simulink model "quadrotor_3dof_fas1"  (R2024a)
settings: Solver=VariableStepAuto  StartTime=0.0  StopTime=20  FixedStep=0.0025  RelTol=1e-3
settings Model: SimulationMode=accelerator  Creator=Dell  LastModifiedBy=44915
settings RTWCC: GPUComputeCapability=3.5

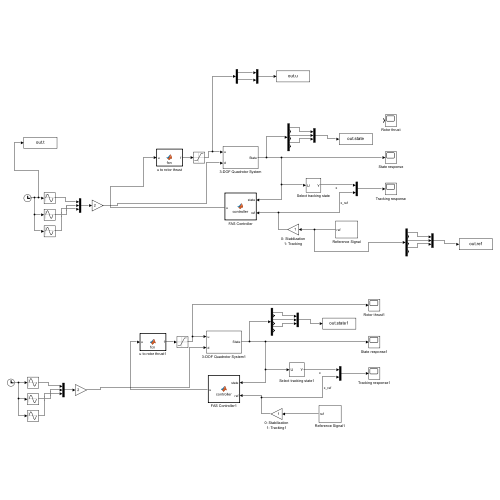
[thumbnail: Simulink's stored preview of the top-level diagram]
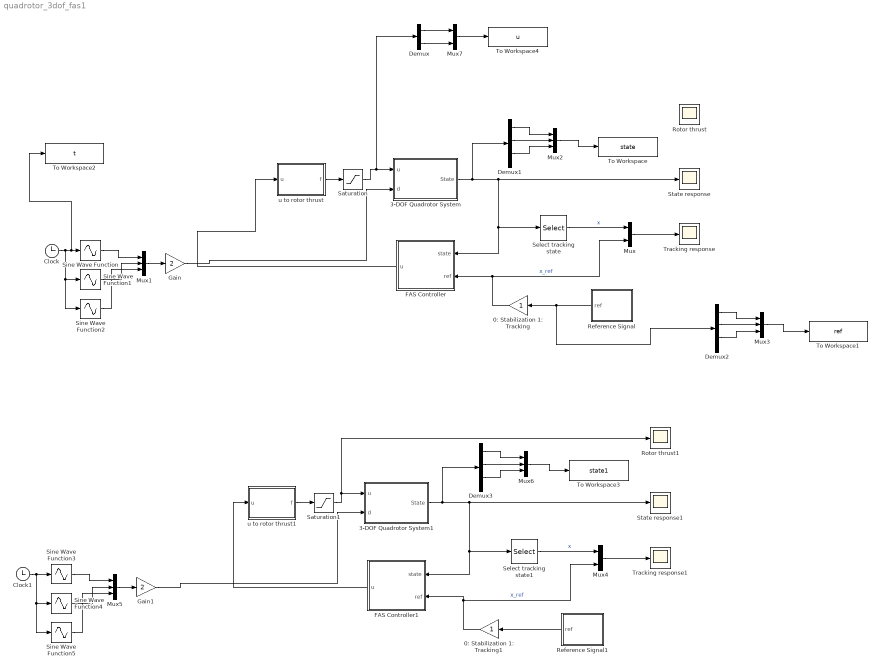
== system quadrotor_3dof_fas1 ==
  0: Stabilization 1: Tracking : Gain
  0: Stabilization 1: Tracking1 : Gain
  3-DOF Quadrotor System : Subsystem
  3-DOF Quadrotor System1 : Subsystem
  Clock : Clock
  Clock1 : Clock
  Demux : Demux  Outputs=2
  Demux1 : Demux  Outputs=6
  Demux2 : Demux  Outputs=6
  Demux3 : Demux  Outputs=6
  FAS Controller : MATLAB Function  TreatAsAtomicUnit=on
  FAS Controller1 : MATLAB Function  TreatAsAtomicUnit=on
  Gain : Gain  Gain=2
  Gain1 : Gain  Gain=2
  Mux : Mux  Inputs=2
  Mux{1..3,5..6} (5 alike) : Mux  Inputs=3
  Mux4 : Mux  Inputs=2
  Mux7 : Mux  Inputs=2
  Reference Signal : Subsystem
  Reference Signal1 : Subsystem
  Rotor thrust : Scope
  Rotor thrust1 : Scope
  Saturation : Saturate  UpperLimit=50  LowerLimit=-50
  Saturation1 : Saturate  UpperLimit=50  LowerLimit=-50
  Select tracking state : Selector  InputPortWidth=6  IndexOptions=Index vector (dialog)  Indices=[1]  OutputSizes=1
  Select tracking state1 : Selector  InputPortWidth=6  IndexOptions=Index vector (dialog)  Indices=[1]  OutputSizes=1
  Sine Wave Function{,1..5} (6 alike) : Sin  TimeSource=Use external signal  Amplitude=0.01  SampleTime=0
  State response : Scope
  State response1 : Scope
  To Workspace : ToWorkspace  VariableName=state  SampleTime=-1
  To Workspace1 : ToWorkspace  VariableName=ref  SampleTime=-1
  To Workspace2 : ToWorkspace  VariableName=t  SampleTime=-1
  To Workspace3 : ToWorkspace  VariableName=state1  SampleTime=-1
  To Workspace4 : ToWorkspace  VariableName=u  SampleTime=-1
  Tracking response : Scope
  Tracking response1 : Scope
  u to rotor thrust : MATLAB Function  TreatAsAtomicUnit=on
  u to rotor thrust1 : MATLAB Function  TreatAsAtomicUnit=on
  wires:
  3-DOF Quadrotor System/1(State) -> Demux1/1, State response/1, Select tracking state/1, FAS Controller/1(state)
  u to rotor thrust/1(f) -> Saturation/1
  Select tracking state/1 -> Mux/1  "x"
  Mux/1 -> Tracking response/1
  0: Stabilization 1: Tracking/1 -> Mux/2, FAS Controller/2(ref)  "x_ref"
  Reference Signal/1(ref) -> Demux2/1, 0: Stabilization 1: Tracking/1
  Saturation/1 -> Demux/1, 3-DOF Quadrotor System/1(u)
  Clock/1 -> Sine Wave Function2/1, Sine Wave Function1/1, To Workspace2/1, Sine Wave Function/1
  Sine Wave Function/1 -> Mux1/1
  Sine Wave Function1/1 -> Mux1/2
  Sine Wave Function2/1 -> Mux1/3
  Mux1/1 -> Gain/1
  Demux1/1 -> Mux2/1
  Demux1/3 -> Mux2/2
  Demux1/5 -> Mux2/3
  Mux2/1 -> To Workspace/1
  Demux2/3 -> Mux3/2
  Demux2/5 -> Mux3/3
  Demux2/1 -> Mux3/1
  Mux3/1 -> To Workspace1/1
  Gain/1 -> 3-DOF Quadrotor System/2(d)
  Mux5/1 -> Gain1/1
  0: Stabilization 1: Tracking1/1 -> Mux4/2, FAS Controller1/2(ref)  "x_ref"
  Demux3/5 -> Mux6/3
  Mux6/1 -> To Workspace3/1
  Demux3/1 -> Mux6/1
  Clock1/1 -> Sine Wave Function5/1, Sine Wave Function4/1, Sine Wave Function3/1
  Sine Wave Function4/1 -> Mux5/2
  u to rotor thrust1/1(f) -> Saturation1/1
  Reference Signal1/1(ref) -> 0: Stabilization 1: Tracking1/1
  Mux4/1 -> Tracking response1/1
  3-DOF Quadrotor System1/1(State) -> Demux3/1, State response1/1, Select tracking state1/1, FAS Controller1/1(state)
  Demux3/3 -> Mux6/2
  Sine Wave Function3/1 -> Mux5/1
  Sine Wave Function5/1 -> Mux5/3
  Gain1/1 -> 3-DOF Quadrotor System1/2(d)
  Select tracking state1/1 -> Mux4/1  "x"
  FAS Controller1/1(u) -> u to rotor thrust1/1(u)
  Saturation1/1 -> 3-DOF Quadrotor System1/1(u), Rotor thrust1/1
  Mux7/1 -> To Workspace4/1
  Demux/1 -> Mux7/1
  Demux/2 -> Mux7/2
  FAS Controller/1(u) -> u to rotor thrust/1(u)

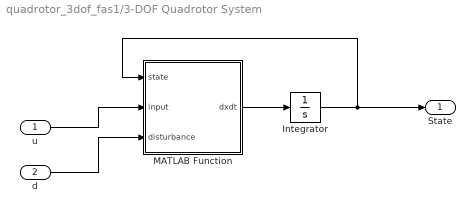
== system quadrotor_3dof_fas1/3-DOF Quadrotor System ==
  u : Inport
  d : Inport  Port=2
  Integrator : Integrator  InitialCondition=zeros(6,1)
  MATLAB Function : MATLAB Function  TreatAsAtomicUnit=on
  State : Outport
  wires:
  MATLAB Function/1(dxdt) -> Integrator/1
  Integrator/1 -> State/1, MATLAB Function/1(state)
  u/1 -> MATLAB Function/2(input)
  d/1 -> MATLAB Function/3(disturbance)

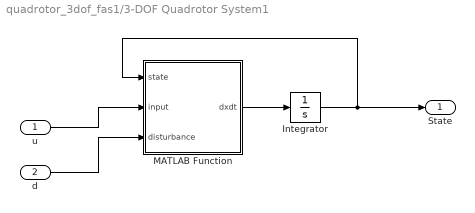
== system quadrotor_3dof_fas1/3-DOF Quadrotor System1 ==
  u : Inport
  d : Inport  Port=2
  Integrator : Integrator  InitialCondition=zeros(6,1)
  MATLAB Function : MATLAB Function  TreatAsAtomicUnit=on
  State : Outport
  wires:
  MATLAB Function/1(dxdt) -> Integrator/1
  Integrator/1 -> State/1, MATLAB Function/1(state)
  u/1 -> MATLAB Function/2(input)
  d/1 -> MATLAB Function/3(disturbance)

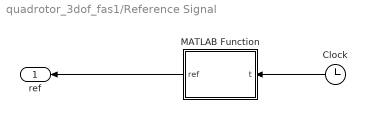
== system quadrotor_3dof_fas1/Reference Signal ==
  Clock : Clock
  MATLAB Function : MATLAB Function  TreatAsAtomicUnit=on
  ref : Outport
  wires:
  Clock/1 -> MATLAB Function/1(t)
  MATLAB Function/1(ref) -> ref/1

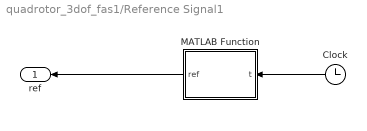
== system quadrotor_3dof_fas1/Reference Signal1 ==
  Clock : Clock
  MATLAB Function : MATLAB Function  TreatAsAtomicUnit=on
  ref : Outport
  wires:
  Clock/1 -> MATLAB Function/1(t)
  MATLAB Function/1(ref) -> ref/1

== matlab function quadrotor_3dof_fas1/3-DOF Quadrotor System1/MATLAB Function ==
  data: state input; input input; dxdt output; disturbance input
function dxdt = quadrotor(state,input,disturbance)
d1=disturbance(1);
d2=disturbance(2);
d3=disturbance(2);
x = state(1);
dx = state(2);
z = state(3);
dz = state(4);
theta = state(5);
dtheta = state(6);
f1 = input(1);
f2 = input(2);
m = 1;
J = 0.01;
g = 9.81;
dxdt = [dx;
        (f1 + f2)/m * sin(theta)+d1;
        dz;
        (f1 + f2)/m * cos(theta) - g+d2;
        dtheta;
        (f2 - f1)/J]+d3;
end

== matlab function quadrotor_3dof_fas1/3-DOF Quadrotor System/MATLAB Function ==
  data: state input; input input; dxdt output; disturbance input
function dxdt = quadrotor(state,input,disturbance)
d1=disturbance(1);
d2=disturbance(2);
d3=disturbance(2);
x = state(1);
dx = state(2);
z = state(3);
dz = state(4);
theta = state(5);
dtheta = state(6);
f1 = input(1);
f2 = input(2);
m = 1;
J = 0.01;
g = 9.81;
dxdt = [dx;
        (f1 + f2)/m * sin(theta)+d1;
        dz;
        (f1 + f2)/m * cos(theta) - g+d2;
        dtheta;
        (f2 - f1)/J]+d3;
end

== matlab function quadrotor_3dof_fas1/Reference Signal/MATLAB Function ==
  data: t input; ref output
function ref = fcn(t)
ref = zeros(6,1);
ref(1) = sin(t);%x
ref(2) = cos(t);%dx
ref(3) = cos(t);%z
ref(4) = -sin(t);%dz
ref(5) = 0;
ref(6) = 0;

== matlab function quadrotor_3dof_fas1/FAS Controller ==
  data: state input; u output; ref input
function u = controller(state,ref)
x = state(1) - ref(1);
dx = state(2) - ref(2);
z = state(3) - ref(3);
dz = state(4) - ref(4);
theta = state(5);
dtheta = state(6) ;

m = 1;
J = 0.01;
g = 9.81;

z1 = x;
z21 = z;
z22 = theta;
dz22 = dtheta;
% Controller gains
A1 = [7.5 19.25 17.75 7]; % more powerful gain

A2 = [1.5 2.5]; % more powerful gain
P1L = 1.0e+05 *[0.5088    1.0093    0.6488    0.1367]*1; 
P2L = 1.0e+01 *[3.2347    2.7086]*0.1; 
z21_d01 = [z; dz];
F=g - A2*z21_d01-2.5*P2L*z21_d01-ref(3);

% F1=g - A2*z21_d01;

u1 = (F) / cos(z22);
ddz = u1 * cos(theta) - g+ref(3);
z21_d12 = [dz; ddz];
dF=-A2*z21_d12-2.5*P2L*z21_d12-ref(4);
du1 = (dF*cos(z22) +F*dz22*sin(z22)) / cos(z22)^2;
d3z = du1*cos(theta) - u1*dtheta*sin(theta)-ref(3);
z21_d23 = [ddz; d3z];
ddF=-A2*z21_d23-2.5*P2L*z21_d23+ref(3);
ddx = u1*sin(theta)+ref(1);
d3x = du1*sin(theta) + u1*dtheta*cos(theta)+ref(2);
z1_d03 = [x; dx; ddx; d3x];


c1 = -u1*cos(z22)^3 -F*sin(z22)^2;
u2_1 = ( ddF*cos(z22)  +F*dz22^2*cos(z22) )*sin(z22);
u2_2 = 2*dz22*sin(z22)*(dF*cos(z22) +F*dz22*sin(z22))/cos(z22);
u2_3 = 2*du1*dz22*cos(z22)^3 - dz22^2*u1*sin(z22)*cos(z22)^2 + A1*z1_d03*cos(z22)^2-ref(1)*cos(z22)^2+0.1*P1L*z1_d03;
u2 = c1 \ (u2_1 + u2_2 + u2_3);

u = [u1; u2];
end

== matlab function quadrotor_3dof_fas1/FAS Controller1 ==
  data: state input; u output; ref input
function u = controller(state,ref)
x = state(1) - ref(1);
dx = state(2) - ref(2);
z = state(3) - ref(3);
dz = state(4) - ref(4);
theta = state(5);
dtheta = state(6) ;

m = 1;
J = 0.01;
g = 9.81;

z1 = x;
z21 = z;
z22 = theta;
dz22 = dtheta;
% Controller gains
A1 = [7.5 19.25 17.75 7]; % more powerful gain

A2 = [1.5 2.5]; % more powerful gain
P1L = 1.0e+05 *[0.5088    1.0093    0.6488    0.1367]*0; 
P2L = 1.0e+01 *[3.2347    2.7086]*0.1*0; 
z21_d01 = [z; dz];
F=g - A2*z21_d01-2.5*P2L*z21_d01-ref(3);

% F1=g - A2*z21_d01;

u1 = (F) / cos(z22);
ddz = u1 * cos(theta) - g+ref(3);
z21_d12 = [dz; ddz];
dF=-A2*z21_d12-2.5*P2L*z21_d12-ref(4);
du1 = (dF*cos(z22) +F*dz22*sin(z22)) / cos(z22)^2;
d3z = du1*cos(theta) - u1*dtheta*sin(theta)-ref(3);
z21_d23 = [ddz; d3z];
ddF=-A2*z21_d23-2.5*P2L*z21_d23+ref(3);
ddx = u1*sin(theta)+ref(1);
d3x = du1*sin(theta) + u1*dtheta*cos(theta)+ref(2);
z1_d03 = [x; dx; ddx; d3x];


c1 = -u1*cos(z22)^3 -F*sin(z22)^2;
u2_1 = ( ddF*cos(z22)  +F*dz22^2*cos(z22) )*sin(z22);
u2_2 = 2*dz22*sin(z22)*(dF*cos(z22) +F*dz22*sin(z22))/cos(z22);
u2_3 = 2*du1*dz22*cos(z22)^3 - dz22^2*u1*sin(z22)*cos(z22)^2 + A1*z1_d03*cos(z22)^2-ref(1)*cos(z22)^2+0.1*P1L*z1_d03;
u2 = c1 \ (u2_1 + u2_2 + u2_3);

u = [u1; u2];
end

== matlab function quadrotor_3dof_fas1/u to rotor thrust ==
  data: u input; f output
function f = fcn(u)
m = 1;
J = 0.01;
g = 9.81;
f1 = (m*u(1) - J*u(2)) / 2;
f2 = m*u(1) - f1;
f = [f1; f2];

== matlab function quadrotor_3dof_fas1/Reference Signal1/MATLAB Function ==
  data: t input; ref output
function ref = fcn(t)
ref = zeros(6,1);
ref(1) = sin(t);%x
ref(2) = cos(t);%dx
ref(3) = cos(t);%z
ref(4) = -sin(t);%dz
ref(5) = 0;
ref(6) = 0;

== matlab function quadrotor_3dof_fas1/u to rotor thrust1 ==
  data: u input; f output
function f = fcn(u)
m = 1;
J = 0.01;
g = 9.81;
f1 = (m*u(1) - J*u(2)) / 2;
f2 = m*u(1) - f1;
f = [f1; f2];
